simulink model "RabinovichFabrikant"  (R2014b)
settings: Solver=ode45  StartTime=0.0  StopTime=10.0  RelTol=1e-3
values from neighbouring files (symbols this model uses):
  a = 0.95    [Run_Aizawa.m]    (also in Run_Arneodo.m = -5.5; Run_Chen.m = 33; Run_Chua.m = 15.6; Run_Chua_4D.m = 0.03)
  g = 0.65    [Run_Aizawa.m]    (also in Run_RabinovichFabrikant.m = 0.09)
undefined symbols (not defined in the file or in its folder): param
settings Model: Creator=Arek  LastModifiedBy=Arek

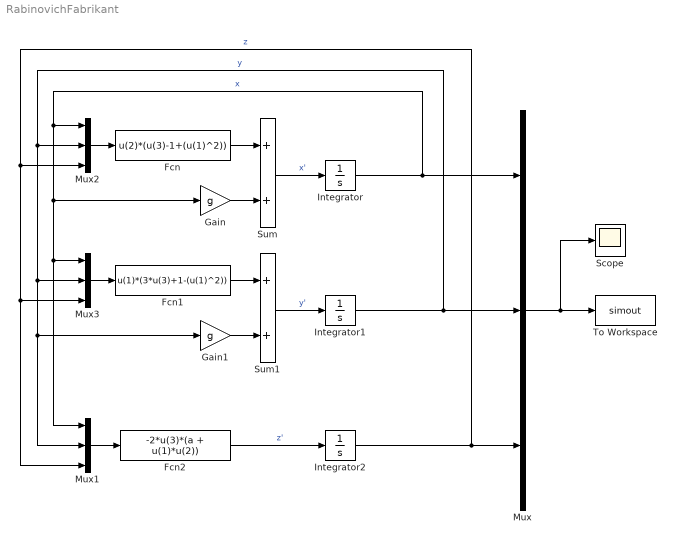
== system RabinovichFabrikant ==
  Fcn : Fcn  Expr=u(2)*(u(3)-1+(u(1)^2))
  Fcn1 : Fcn  Expr=u(1)*(3*u(3)+1-(u(1)^2))
  Fcn2 : Fcn  Expr=-2*u(3)*(a + u(1)*u(2))
  Gain : Gain  Gain=g
  Gain1 : Gain  Gain=g
  Integrator : Integrator  InitialCondition=param.ic(1)
  Integrator1 : Integrator  InitialCondition=param.ic(2)
  Integrator2 : Integrator  InitialCondition=param.ic(3)
  Mux{,1..3} (4 alike) : Mux  Inputs=3
  Scope : Scope
      settings: ShowLegends=on
  Sum : Sum
  Sum1 : Sum
  To Workspace : ToWorkspace  VariableName=simout  SaveFormat=Timeseries  SampleTime=-1
  wires:
  Integrator/1 -> Mux2/1, Gain/1, Mux1/1, Mux3/1, Mux/1  "x"
  Sum1/1 -> Integrator1/1  "y'"
  Integrator1/1 -> Mux3/2, Mux1/2, Gain1/1, Mux2/2, Mux/2  "y"
  Fcn2/1 -> Integrator2/1  "z'"
  Integrator2/1 -> Mux2/3, Mux1/3, Mux3/3, Mux/3  "z"
  Mux/1 -> Scope/1, To Workspace/1
  Sum/1 -> Integrator/1  "x'"
  Mux2/1 -> Fcn/1
  Mux3/1 -> Fcn1/1
  Gain/1 -> Sum/2
  Fcn/1 -> Sum/1
  Gain1/1 -> Sum1/2
  Fcn1/1 -> Sum1/1
  Mux1/1 -> Fcn2/1
